simulink model "model_min_mine"  (R2018a)
settings: Solver=ode45  StartTime=0.0  StopTime=20  RelTol=1e-3
(part 10 of 10)

== system model_min_mine/5 систем підйому/6/6-періодні/6-ти періодна пр/Допоміжний1/Генераці ==
  In1 : Inport
  Trigger : TriggerPort  TriggerType=either  VariantControl=(inherit)  ShowOutputPort=on
  Out1 : Outport
  wires:
  In1/1 -> Out1/1

== system model_min_mine/5 систем підйому/6/7-періодні/7-ми періодна криволінійна/Subsystem/Генераці ==
  In1 : Inport
  Trigger : TriggerPort  TriggerType=either  VariantControl=(inherit)  ShowOutputPort=on
  Out1 : Outport
  wires:
  In1/1 -> Out1/1

== system model_min_mine/5 систем підйому/6/7-періодні/7-ми періодна криволінійна/Subsystem3/Генераці ==
  In1 : Inport
  Trigger : TriggerPort  TriggerType=either  VariantControl=(inherit)  ShowOutputPort=on
  Out1 : Outport
  wires:
  In1/1 -> Out1/1

== system model_min_mine/5 систем підйому/6/7-періодні/7-ми періодна криволінійна/Subsystem6/Генераці ==
  In1 : Inport
  Trigger : TriggerPort  TriggerType=either  VariantControl=(inherit)  ShowOutputPort=on
  Out1 : Outport
  wires:
  In1/1 -> Out1/1

== system model_min_mine/5 систем підйому/6/7-періодні/7-ми періодна криволінійна/Допоміжний/Генераці ==
  In1 : Inport
  Trigger : TriggerPort  TriggerType=either  VariantControl=(inherit)  ShowOutputPort=on
  Out1 : Outport
  wires:
  In1/1 -> Out1/1

== system model_min_mine/5 систем підйому/6/7-періодні/7-ми періодна криволінійна/Допоміжний1/Генераці ==
  In1 : Inport
  Trigger : TriggerPort  TriggerType=either  VariantControl=(inherit)  ShowOutputPort=on
  Out1 : Outport
  wires:
  In1/1 -> Out1/1

== system model_min_mine/5 систем підйому/6/7-періодні/7-ми періодна пр/Subsystem/Генераці ==
  In1 : Inport
  Trigger : TriggerPort  TriggerType=either  VariantControl=(inherit)  ShowOutputPort=on
  Out1 : Outport
  wires:
  In1/1 -> Out1/1

== system model_min_mine/5 систем підйому/6/7-періодні/7-ми періодна пр/Subsystem1/Генераці ==
  In1 : Inport
  Trigger : TriggerPort  TriggerType=either  VariantControl=(inherit)  ShowOutputPort=on
  Out1 : Outport
  wires:
  In1/1 -> Out1/1

== system model_min_mine/5 систем підйому/6/7-періодні/7-ми періодна пр/Subsystem2/Генераці ==
  In1 : Inport
  Trigger : TriggerPort  TriggerType=either  VariantControl=(inherit)  ShowOutputPort=on
  Out1 : Outport
  wires:
  In1/1 -> Out1/1

== system model_min_mine/5 систем підйому/6/7-періодні/7-ми періодна пр/Subsystem3/Генераці ==
  In1 : Inport
  Trigger : TriggerPort  TriggerType=either  VariantControl=(inherit)  ShowOutputPort=on
  Out1 : Outport
  wires:
  In1/1 -> Out1/1

== system model_min_mine/5 систем підйому/6/7-періодні/7-ми періодна пр/Subsystem6/Генераці ==
  In1 : Inport
  Trigger : TriggerPort  TriggerType=either  VariantControl=(inherit)  ShowOutputPort=on
  Out1 : Outport
  wires:
  In1/1 -> Out1/1

== system model_min_mine/5 систем підйому/6/7-періодні/7-ми періодна пр/Допоміжний/Генераці ==
  In1 : Inport
  Trigger : TriggerPort  TriggerType=either  VariantControl=(inherit)  ShowOutputPort=on
  Out1 : Outport
  wires:
  In1/1 -> Out1/1

== system model_min_mine/5 систем підйому/6/7-періодні/7-ми періодна пр/Допоміжний1/Генераці ==
  In1 : Inport
  Trigger : TriggerPort  TriggerType=either  VariantControl=(inherit)  ShowOutputPort=on
  Out1 : Outport
  wires:
  In1/1 -> Out1/1
